simulink model "CSTRsimple"  (R2018a)
settings: Solver=VariableStepAuto  StartTime=0.0  StopTime=10.0  RelTol=1e-3
settings Model: Creator=Mahe  LastModifiedBy=Mahe

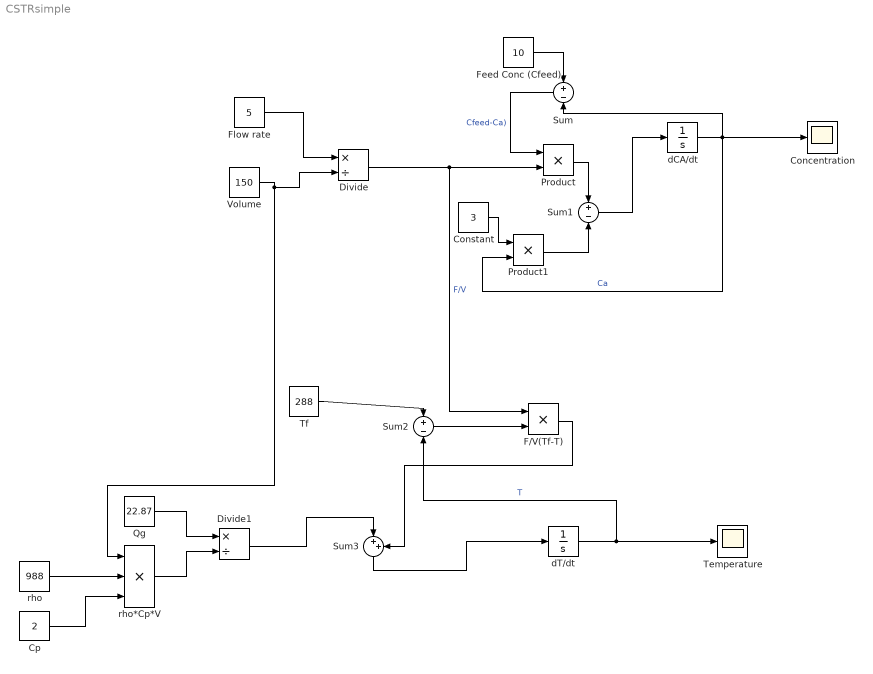
== system CSTRsimple ==
  Concentration : Scope
  Constant : Constant  Value=3
  Cp : Constant  Value=2
  Divide : Product  Inputs=*/
  Divide1 : Product  Inputs=*/
  F/V(Tf-T) : Product
  Feed Conc (Cfeed) : Constant  Value=10
  Flow rate : Constant  Value=5
  Product : Product
  Product1 : Product
  Qg : Constant  Value=22.87
  Sum : Sum  Inputs=+-
  Sum1 : Sum  Inputs=+-
  Sum2 : Sum  Inputs=+-
  Sum3 : Sum  Inputs=|++
  Temperature : Scope
  Tf : Constant  Value=288
  Volume : Constant  Value=150  VectorParams1D=off
  dCA/dt : Integrator  InitialCondition=100
  dT/dt : Integrator  InitialCondition=250
  rho : Constant  Value=988
  rho*Cp*V : Product  Inputs=3
  wires:
  Flow rate/1 -> Divide/1
  Volume/1 -> rho*Cp*V/1, Divide/2
  dCA/dt/1 -> Product1/2, Concentration/1, Sum/2  "Ca"
  Feed Conc (Cfeed)/1 -> Sum/1
  Divide/1 -> F/V(Tf-T)/1, Product/2  "F/V"
  Sum/1 -> Product/1  "Cfeed-Ca)"
  Product/1 -> Sum1/1
  Product1/1 -> Sum1/2
  Constant/1 -> Product1/1
  Sum1/1 -> dCA/dt/1
  dT/dt/1 -> Sum2/2, Temperature/1  "T"
  Tf/1 -> Sum2/1
  Sum2/1 -> F/V(Tf-T)/2
  Cp/1 -> rho*Cp*V/3
  rho/1 -> rho*Cp*V/2
  rho*Cp*V/1 -> Divide1/2
  Qg/1 -> Divide1/1
  Divide1/1 -> Sum3/1
  F/V(Tf-T)/1 -> Sum3/2
  Sum3/1 -> dT/dt/1
